simulink model "week1_2"  (R2020b)
settings: Solver=VariableStepAuto  StartTime=0.0  StopTime=100  RelTol=1e-3
undefined symbols (not defined in the file): b, K1, K2, M1, M2
settings Model: Creator=Lenovo  LastModifiedBy=Lenovo

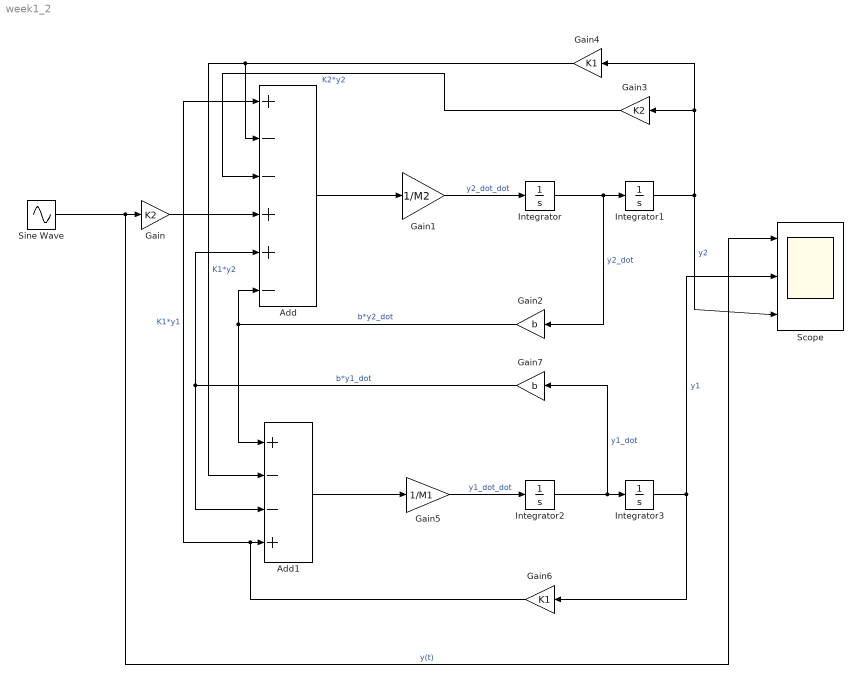
== system week1_2 ==
  Add : Sum  Inputs=+--++-
  Add1 : Sum  Inputs=+--+
  Gain : Gain  Gain=K2
  Gain1 : Gain  Gain=1/M2
  Gain2 : Gain  Gain=b
  Gain3 : Gain  Gain=K2
  Gain4 : Gain  Gain=K1
  Gain5 : Gain  Gain=1/M1
  Gain6 : Gain  Gain=K1
  Gain7 : Gain  Gain=b
  Integrator{,1..3} (4 alike) : Integrator
  Scope : Scope  NumInputPorts=3
  Sine Wave : Sin  Amplitude=2  SampleTime=0
  wires:
  Sine Wave/1 -> Scope/1, Gain/1  "y(t)"
  Gain/1 -> Add/4
  Add/1 -> Gain1/1
  Gain1/1 -> Integrator/1  "y2_dot_dot"
  Integrator/1 -> Gain2/1, Integrator1/1  "y2_dot"
  Gain2/1 -> Add/6, Add1/1  "b*y2_dot"
  Integrator1/1 -> Scope/3, Gain4/1, Gain3/1  "y2"
  Gain4/1 -> Add1/2, Add/2  "K1*y2"
  Gain3/1 -> Add/3  "K2*y2"
  Add1/1 -> Gain5/1
  Gain5/1 -> Integrator2/1  "y1_dot_dot"
  Integrator2/1 -> Gain7/1, Integrator3/1  "y1_dot"
  Gain7/1 -> Add1/3, Add/5  "b*y1_dot"
  Integrator3/1 -> Scope/2, Gain6/1  "y1"
  Gain6/1 -> Add/1, Add1/4  "K1*y1"
